simulink model "sm_car_harness_body_to_world"  (R2019a)
settings: Solver=VariableStepAuto  StartTime=0.0  StopTime=10.0  MaxStep=0.01  RelTol=1e-3
libraries: sm_lib x3, sm_car_lib x2, Body x1
Description:
  | Copyright 2020 The MathWorks, Inc.
settings Model: Creator=smiller  LastModifiedBy=smiller
settings DataIOCC: ReturnWorkspaceOutputs=off
settings DebuggingCC: PregeneratedLibrarySubsystemCodeDiagnostic=none  ArithmeticOperatorsInVariantConditions=warning
settings SFSimCC: SimUseLocalCustomCode=off
settings RTWCC: RTWUseLocalCustomCode=off
settings DiagnosticsConfigSet: SimMechanicsConflictingReferenceFrames=none
settings ExplorerConfigSet: InternalSimMechanicsExplorerSettings="<ExplorerConfiguration><canonicalview>default</canonicalview><AnimationSetting><BasePlaybackSpeed>1.0</BasePlaybackSpeed><PlaybackSpeedFactor>1.0</PlaybackSpeedFactor></AnimationSetting><TilePanel><TileInfo><Tiles Columns=\"2\" Count=\"4\" Rows=\"2\"><Column Weight=\"0.4993\"/><Column Weight=\"0.5007\"/><Row Weight=\"0.4992\"/><Row Weight=\"0.5008\"/><Tile Height=\"1\" Width=\"1\" X=\"0\" Y=\"0\"/><Tile Height=\"1\" Width=\"1\" X=\"0\" Y=\"1\"/><Tile Height=\"1\" Width=\"1\" X=\"1\" Y=\"0\"/><Tile Height=\"1\" Width=\"1\" X=\"1\" Y=\"1\"/></Tiles></TileInfo><SceneInfo><SceneViewer><BGColor><R>1</R><G>1</G><B>1</B></BGColor><Camera><DoPerspective>off</DoPerspective><Position><X>-101.838946705900781</X><Y>-283.63123193047511</Y><Z>0.64011586973833845</Z></Position><Center><X>-101.838946705900781</X><Y>-6.41538014201081808e-06</Y><Z>0.64011586973833845</Z></Center><Up><X>0</X><Y>-0</Y><Z>1</Z></Up><ViewLimDist>1</ViewLimDist><YLim>2.86761968108461085</YLim><XLim>2.99152917347715563</XLim></Camera></SceneViewer><SceneViewer><BGColor><R>1</R><G>1</G><B>1</B></BGColor><Camera><DoPerspective>off</DoPerspective><Position><X>-101.803495962212878</X><Y>0.45246930792062301</Y><Z>285.653405729638393</Z></Position><Center><X>-101.803495962212878</X><Y>0.45246930792062301</Y><Z>0.782626499049598578</Z></Center><Up><X>0</X><Y>1</Y><Z>-0</Z></Up><ViewLimDist>1</ViewLimDist><YLim>4.67017961555967975</YLim><XLim>4.8569868001820673</XLim></Camera></SceneViewer><SceneViewer><BGColor><R>1</R><G>1</G><B>1</B></BGColor><Camera><DoPerspective>off</DoPerspective><Position><X>283.631232019339791</X><Y>-0.171702046803467567</Y><Z>0.790728238821008844</Z></Position><Center><X>-2.47108863504763576e-06</X><Y>-0.171702046803467567</Y><Z>0.790728238821008844</Z></Center><Up><X>-0</X><Y>0</Y><Z>1</Z></Up><ViewLimDist>1</ViewLimDist><YLim>3.10488434625603471</YLim><XLim>3.24862899191603605</XLim></Camera></SceneViewer><SceneViewer><BGColor><R>1</R><G>1</G><B>1</B></BGColor><Camera><DoPerspective>off</DoPerspective><Position><X>95.3157018406999441</X><Y>-197.716862101705203</Y><Z>197.684422216712676</Z></Position><Center><X>-68.2566092783274883</X><Y>-34.1445509826777922</Y><Z>34.1121110976852435</Z></Center><Up><X>-0.408248290463863073</X><Y>0.408248290463863073</Y><Z>0.816496580927726145</Z></Up><ViewLimDist>1</ViewLimDist><YLim>4.91424145113695321</YLim><XLim>5.12593185210900604</XLim></Camera></SceneViewer></SceneInfo></TilePanel><MechEditorPanel><Cameras/><GfxPanelCameraMap/><VideoCreator><PlaybackSpeedRatio>1.0</PlaybackSpeedRatio><FrameRate>30</FrameRate><VideoFormat>Motion JPEG AVI</VideoFormat><FrameSize>auto</FrameSize></VideoCreator></MechEditorPanel></ExplorerConfiguration>"

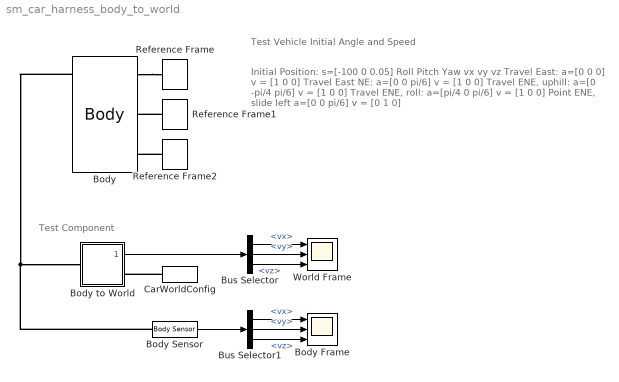
== system sm_car_harness_body_to_world ==
  note: Initial Position: s=[-100 0 0.05]
      | Roll Pitch Yaw vx vy vz
      | Travel East: a=[0 0 0] v = [1 0 0]
      | Travel East NE: a=[0 0 pi/6] v = [1 0 0]
      | Travel ENE, uphill: a=[0 -pi/4 pi/6] v = [1 0 0]
      | Travel ENE, roll: a=[pi/4 0 pi/6] v = [1 0 0]
      | Point ENE, slide left a=[0 0 pi/6] v = [0 1 0]
  note: Test Component
  note: Test Vehicle Initial Angle and Speed
  Body : Body/Body  hp_mount_fa=Vehicle.Chassis.Body.sAxleF.Value  hp_mount_ra=Vehicle.Chassis.Body.sAxleR.Value  hp_mount_power=Vehicle.Chassis.Body.sPower.Value  hp_chassis_cg=Vehicle.Chassis.Body.sCG.Value  hp_mount_hitchr=Vehicle.Chassis.Body.sHitchR.Value  chassis_mass=Vehicle.Chassis.Body.m.Value  chassis_inertia=Vehicle.Chassis.Body.J.Value  clr_chassis_hp_cg=Visual.hp.clr  opc_chassis_hp_cg=Visual.hp.opc  size_chassis_hp_cg=Visual.hp.rad  BodyGeometry=Chassis.Body.BodyGeometry  Passenger=Vehicle.Chassis.Body.Passenger  InitTriggerDropdown=0
  Body Frame : Scope  NumInputPorts=3
  Body Sensor : sm_car_lib/Sensors/Body Sensor  SystemSampleTime=-1
  Body to World : Subsystem  Tag=__SL_testing_harness_stub_
  Bus Selector : BusSelector  OutputSignals=vx,vy,vz
  Bus Selector1 : BusSelector  OutputSignals=vx,vy,vz
  CarWorldConfig : sm_car_lib/Environment/CarWorldConfig  UseLocalSolver=off  LocalSolverChoice=Backward Euler  LocalSolverSampleTime=0.005  DoFixedCost=off  MaxNonlinIter=3  popup_scene=Road Two Lane  GravityVector=[0 0 0]
  Reference Frame : sm_lib/Frames and Transforms/Reference Frame
  Reference Frame1 : sm_lib/Frames and Transforms/Reference Frame
  Reference Frame2 : sm_lib/Frames and Transforms/Reference Frame
  World Frame : Scope  NumInputPorts=3
  wires:
  Body to World/1(harness_out_1) -> Bus Selector/1
  Bus Selector/1 -> World Frame/1  "<vx>"
  Bus Selector/2 -> World Frame/2  "<vy>"
  Bus Selector/3 -> World Frame/3  "<vz>"
  Bus Selector1/3 -> Body Frame/3  "<vz>"
  Bus Selector1/2 -> Body Frame/2  "<vy>"
  Bus Selector1/1 -> Body Frame/1  "<vx>"
  Body Sensor/1 -> Bus Selector1/1
  connections:
  Body/LConn1 -- Body Sensor/LConn1 -- Body to World/LConn1
  CarWorldConfig/RConn1 -- Body to World/RConn1
  Body/RConn1 -- Reference Frame/RConn1
  Reference Frame1/RConn1 -- Body/RConn2
  Reference Frame2/RConn1 -- Body/RConn3

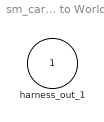
== system sm_car_harness_body_to_world/Body to World ==
  harness_out_1 : Outport
